simulink model "project5"  (R2020b)
settings: Solver=VariableStepAuto  StartTime=0.0  StopTime=10.0  RelTol=1e-3
settings Model: Creator=shrin  LastModifiedBy=shrin

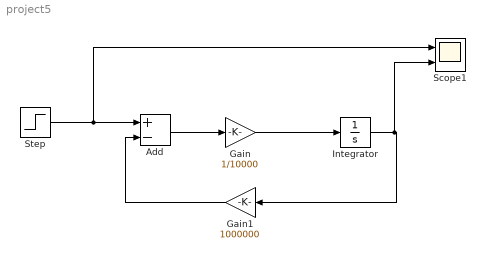
== system project5 ==
  Add : Sum  Inputs=+-
  Gain : Gain  Gain=1/10000
  Gain1 : Gain  Gain=1000000
  Integrator : Integrator
  Scope1 : Scope  NumInputPorts=2
  Step : Step  SampleTime=0
  wires:
  Add/1 -> Gain/1
  Gain/1 -> Integrator/1
  Gain1/1 -> Add/2
  Step/1 -> Scope1/1, Add/1
  Integrator/1 -> Scope1/2, Gain1/1
